simulink model "assignment_1a"  (R2023b)
settings: Solver=ode4  StartTime=0.0  StopTime=10.0  FixedStep=0.001  RelTol=1e-3
settings Model: Creator=HP  LastModifiedBy=HP

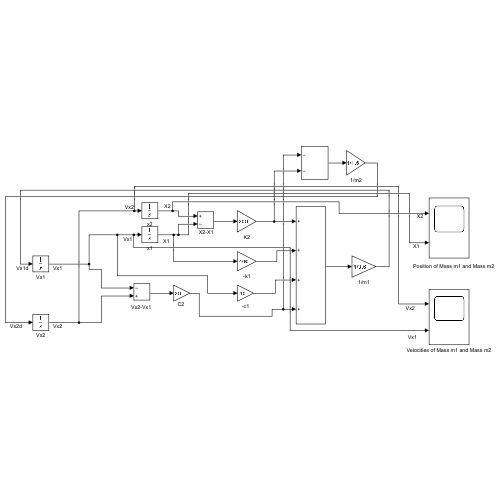
[thumbnail: Simulink's stored preview of the top-level diagram]
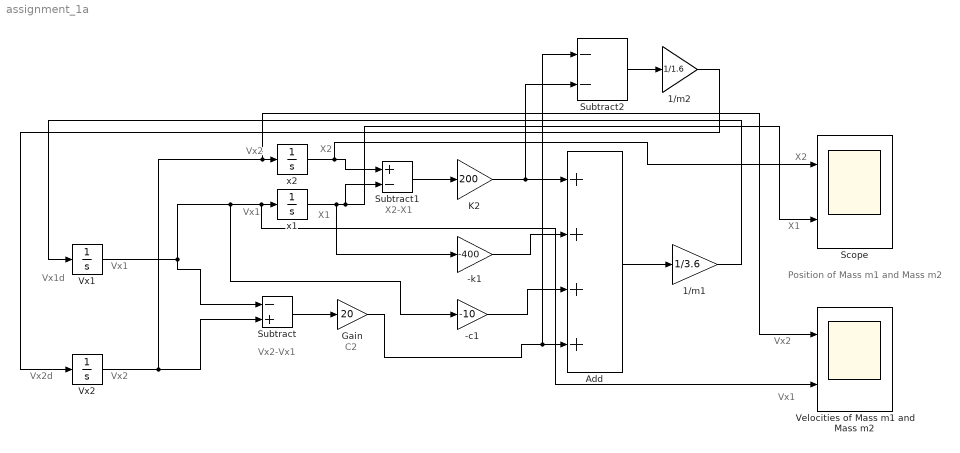
== system assignment_1a ==
  note: Vx2
  note: Vx1
  note: Position of Mass m1 and Mass m2
  note: X1
  note: X2
  note: X2-X1
  note: X2
  note: Vx2
  note: C2
  note: Vx2-Vx1
  note: Vx1d
  note: Vx1
  note: Vx2d
  note: Vx2
  note: X1
  note: Vx1
  -c1 : Gain  Gain=-10
  -k1 : Gain  Gain=-400
  1/m1 : Gain  Gain=1/3.6
  1/m2 : Gain  Gain=1/1.6
  Add : Sum  Inputs=++++
  Gain : Gain  Gain=20
  K2 : Gain  Gain=200
  Scope : Scope  NumInputPorts=2
  Subtract : Sum  Inputs=-+
  Subtract1 : Sum  Inputs=+-
  Subtract2 : Sum  Inputs=--
  Velocities of Mass m1 and Mass m2 : Scope  NumInputPorts=2
  Vx1 : Integrator
  Vx2 : Integrator
  x1 : Integrator  InitialCondition=0.05
  x2 : Integrator  InitialCondition=0.05
  wires:
  1/m1/1 -> Vx1/1
  1/m2/1 -> Vx2/1
  Subtract/1 -> Gain/1
  x1/1 -> Scope/2, Subtract1/2, -k1/1
  Vx1/1 -> Subtract/1, -c1/1, Velocities of Mass m1 and Mass m2/2, x1/1
  Vx2/1 -> Velocities of Mass m1 and Mass m2/1, x2/1, Subtract/2
  x2/1 -> Scope/1, Subtract1/1
  Subtract1/1 -> K2/1
  K2/1 -> Subtract2/2, Add/1
  -k1/1 -> Add/2
  -c1/1 -> Add/3
  Gain/1 -> Subtract2/1, Add/4
  Add/1 -> 1/m1/1
  Subtract2/1 -> 1/m2/1
